simulink model "s0205"  (Simulink 7.0)
settings: Solver=ode3  SolverMode=SingleTasking  StartTime=0.0  StopTime=900  FixedStep=1  MaxStep=1  RelTol=1e-3  AbsTol=1e-6
values from neighbouring files (symbols this model uses):
  t0 = .2    (= 0.2)    [m0203.m]    (also in m0205.m)
  T1 = 3*T1    (= 0.3)    [m0203.m]    (also in m0204.m = 0.1; m0205.m = 0.1; m0207.m = 0.1; m0221d.m = 1/a0)
  ue1 = ue1amp    (= 1)    [m0205.m]
  ue2 = ue2amp    (= -0.5)    [m0205.m]
  ue2par = .3    (= 0.3)    [m0205.m]
settings Model: Creator=froriep  LastModifiedBy=froriep
settings DataIOCC: LimitDataPoints=off  SaveOutput=off  TimeSaveName=t
settings OptimizationCC: BooleanDataType=off  InlineInvariantSignals=on
settings DebuggingCC: SaveWithParameterizedLinksMsg=none  SignalResolutionControl=TryResolveAllWithWarning  SolverPrmCheckMsg=none  MultiTaskDSMMsg=warning  MultiTaskCondExecSysMsg=none  StrictBusMsg=None
settings HardwareCC: TargetUnknown=on
settings RTWCC: IncludeERTFirstTime=on
settings GRTTargetCC: TargetFcnLib=ansi_tfl_tmw.mat  ModelReferenceCompliant=off  MatFileLogging=off

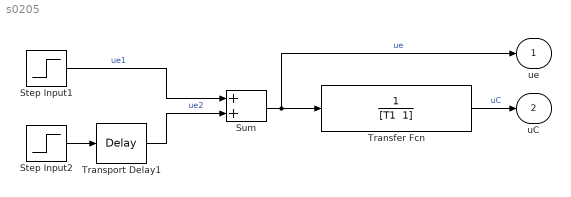
== system s0205 ==
  Step Input1 : Step  Time=t0  After=ue1  SampleTime=0
  Step Input2 : Step  Time=t0  After=ue2  SampleTime=0
  Sum : Sum  OutDataType=sfix(16)  OutScaling=2^0  SaturateOnIntegerOverflow=on  InputSameDT=on
  Transfer Fcn : TransferFcn  Denominator="[T1  1]"
  Transport Delay1 : TransportDelay  DelayTime=ue2par
  ue : Outport  OutDataType=sfix(16)  OutScaling=2^0
  uC : Outport  Port=2  OutDataType=sfix(16)  OutScaling=2^0
  wires:
  Transfer Fcn/1 -> uC/1  "uC"
  Sum/1 -> Transfer Fcn/1, ue/1  "ue"
  Step Input2/1 -> Transport Delay1/1
  Step Input1/1 -> Sum/1  "ue1"
  Transport Delay1/1 -> Sum/2  "ue2"
